simulink model "modelGod"  (R2020b)
settings: Solver=VariableStepAuto  StartTime=0.0  StopTime=50  MaxStep=0.01  RelTol=1e-3
values from neighbouring files (symbols this model uses):
  A = [-Ya_Alpha 1 0 ... (first row only)    [StateSpace.m]    (also in matan.m = [1 -1/p; modelGodPrint.m = figure; print2.m = figure)
  B = [0;Mz_deltaB;0]    [StateSpace.m]    (also in matan.m = [0; -K_v*Vzad/(1/(W*Wpriv)+K_wz)]; modelGodPrint.m = figure)
  C = [1 0 0; 0 1 0; 0 0 1]    [StateSpace.m]    (also in modelGodPrint.m = figure)
  D = [0;0;0]    [StateSpace.m]    (also in modelGodPrint.m = figure)
  K_v = nu*K_wz    [Synthesis_of_ACS.m]    (also in main.m = 2)
  K_wz = e*K_wzGr    [Synthesis_of_ACS.m]    (also in main.m = -2)
libraries: cstblocks x1
settings Model: Creator=User  LastModifiedBy=User

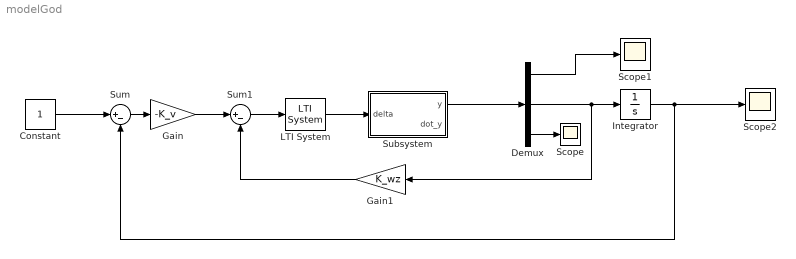
== system modelGod ==
  Constant : Constant
  Demux : Demux  Outputs=3
  Gain : Gain  Gain=-K_v
  Gain1 : Gain  Gain=K_wz
  Integrator : Integrator
  LTI System : cstblocks/LTI System  sys=Drive  IC=[]
  Scope : Scope
  Scope1 : Scope
  Scope2 : Scope
  Subsystem : Subsystem
  Sum : Sum  Inputs=|+-
  Sum1 : Sum  Inputs=|+-
  wires:
  Sum/1 -> Gain/1
  Constant/1 -> Sum/1
  Gain/1 -> Sum1/1
  Sum1/1 -> LTI System/1
  LTI System/1 -> Subsystem/1(delta)
  Subsystem/1(y) -> Demux/1
  Demux/2 -> Gain1/1, Integrator/1
  Gain1/1 -> Sum1/2
  Integrator/1 -> Scope2/1, Sum/2
  Demux/3 -> Scope/1
  Demux/1 -> Scope1/1

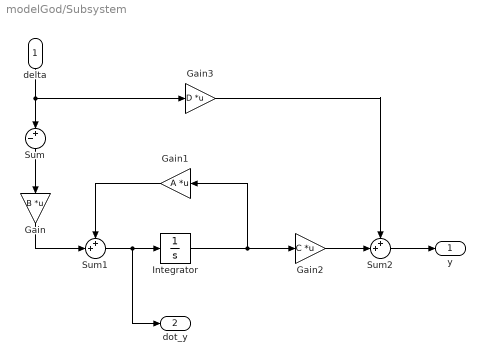
== system modelGod/Subsystem ==
  delta : Inport
  Gain : Gain  Gain=B  Multiplication=Matrix(K*u)
  Gain1 : Gain  Gain=A  Multiplication=Matrix(K*u)
  Gain2 : Gain  Gain=C  Multiplication=Matrix(K*u)
  Gain3 : Gain  Gain=D  Multiplication=Matrix(K*u)
  Integrator : Integrator
  Sum : Sum  Inputs=-+|
  Sum1 : Sum  Inputs=++|
  Sum2 : Sum  Inputs=++|
  y : Outport
  dot_y : Outport  Port=2
  wires:
  Sum/1 -> Gain/1
  delta/1 -> Gain3/1, Sum/2
  Sum1/1 -> dot_y/1, Integrator/1
  Gain/1 -> Sum1/2
  Integrator/1 -> Gain2/1, Gain1/1
  Gain1/1 -> Sum1/1
  Gain2/1 -> Sum2/2
  Sum2/1 -> y/1
  Gain3/1 -> Sum2/1
